simulink model "RBCM_Model"  (R2024b)
settings: Solver=FixedStepAuto  StartTime=0.0  StopTime=10.0  RelTol=1e-3
PreLoadFcn:
  | % NXP_MBDT_S32K3 callback: DO NOT REMOVE
  | mbd_s32k3.common.nxp.model_callbacks.preLoadFcn();
PostLoadFcn:
  | % NXP_MBDT_S32K3 callback: DO NOT REMOVE
  | mbd_s32k3.common.nxp.model_callbacks.postLoadFcn();
InitFcn:
  | % NXP_MBDT_S32K3 callback: DO NOT REMOVE
  | mbd_s32k3.common.nxp.model_callbacks.initFcn();
undefined symbols (not defined in the file or in its folder): AccuFanPwr_hHsd3ch2, BspdPwr_lHsd1ch2, BuzzerPwr_lHsd3ch3, DevicePwr_12v_lHsd1ch1, DevicePwr_hHsd1ch2, DrsPwr_8v_lHsd3ch1, hHsd_Diagnose_AdcBuffer, ILPwr_hHsd1ch1, lHsd_Diagnose_AdcBuffer, LoggerPwr_lHsd1ch3, PumpFan1_hHsd4ch1, PumpFan2_hHsd4ch2, PumpPwr_hHsd3ch1, RGBLED0state, TaillightPwr_lHsd3ch4, TempSensorPwr_lHsd1ch4
libraries: mbd_s32k3_io_library x127, simulink x48, canmsglib x8, mbd_s32k3_communication_library x7, mbd_s32k3_isr_library x6, mbd_s32k3_cdd_library x3, mbd_s32k3_utility_library x1
(part 9 of 10)

== system RBCM_Model/HSD诊断分析子系统/旧模型/HSDh片选执行单元3 ==
  y : Inport
  Data Type Conversion4 : DataTypeConversion  OutDataTypeStr=boolean  SaturateOnIntegerOverflow=off  RndMeth=Floor
  Dio : mbd_s32k3_io_library/Dio  api_func=Dio_WriteChannel  channel=RGBLED0_BLUE  channel_group=No channel groups configured  port=PTB_H  gpioSim=on  text=<binary blob, 15399 chars, not shown>
      settings: SourceProductName=IO Blocks
  wires:
  Data Type Conversion4/1 -> Dio/1
  y/1 -> Data Type Conversion4/1

== system RBCM_Model/HSD诊断分析子系统/旧模型/HSDh片选执行单元4 ==
  y : Inport
  Data Type Conversion4 : DataTypeConversion  OutDataTypeStr=boolean  SaturateOnIntegerOverflow=off  RndMeth=Floor
  Dio : mbd_s32k3_io_library/Dio  api_func=Dio_WriteChannel  channel=RGBLED0_BLUE  channel_group=No channel groups configured  port=PTB_H  gpioSim=on  text=<binary blob, 15399 chars, not shown>
      settings: SourceProductName=IO Blocks
  wires:
  y/1 -> Data Type Conversion4/1
  Data Type Conversion4/1 -> Dio/1

== system RBCM_Model/HSD诊断分析子系统/旧模型/HSDl片选执行单元2 ==
  y : Inport
  Bitwise AND2 : simulink/Logic and Bit Operations/Bitwise Operator  logicop=AND  UseBitMask=on  BitMask=bin2dec('00000001')  BitMaskRealWorld=Stored Integer
      settings: LibrarySourceBlock=|
      | simulink/Quick Insert/Logic and Bit
      | Operations/Bitwise AND
  Bitwise AND3 : simulink/Logic and Bit Operations/Bitwise Operator  logicop=AND  UseBitMask=on  BitMask=bin2dec('00000010')  BitMaskRealWorld=Stored Integer
      settings: LibrarySourceBlock=|
      | simulink/Quick Insert/Logic and Bit
      | Operations/Bitwise AND
  Data Type Conversion : DataTypeConversion  OutDataTypeStr=boolean  SaturateOnIntegerOverflow=off  RndMeth=Floor
  Data Type Conversion1 : DataTypeConversion  OutDataTypeStr=boolean  SaturateOnIntegerOverflow=off  RndMeth=Floor
  Dio : mbd_s32k3_io_library/Dio  api_func=Dio_WriteChannel  channel=RGBLED0_BLUE  channel_group=No channel groups configured  port=PTB_H  gpioSim=on  text=<binary blob, 15399 chars, not shown>
      settings: SourceProductName=IO Blocks
  Dio1 : mbd_s32k3_io_library/Dio  api_func=Dio_WriteChannel  channel=RGBLED0_BLUE  channel_group=No channel groups configured  port=PTB_H  gpioSim=on  text=<binary blob, 15399 chars, not shown>
      settings: SourceProductName=IO Blocks
  Shift Arithmetic1 : ArithShift  BitShiftNumber=1  BitShiftDirection=Right
  Shift Arithmetic2 : ArithShift  BitShiftDirection=Right
  wires:
  Data Type Conversion1/1 -> Dio1/1
  Data Type Conversion/1 -> Dio/1
  y/1 -> Bitwise AND3/1, Bitwise AND2/1
  Shift Arithmetic2/1 -> Data Type Conversion/1
  Bitwise AND3/1 -> Shift Arithmetic1/1
  Bitwise AND2/1 -> Shift Arithmetic2/1
  Shift Arithmetic1/1 -> Data Type Conversion1/1

== system RBCM_Model/HSD诊断分析子系统/旧模型/HSDl片选执行单元3 ==
  y : Inport
  Bitwise AND2 : simulink/Logic and Bit Operations/Bitwise Operator  logicop=AND  UseBitMask=on  BitMask=bin2dec('00000001')  BitMaskRealWorld=Stored Integer
      settings: LibrarySourceBlock=|
      | simulink/Quick Insert/Logic and Bit
      | Operations/Bitwise AND
  Bitwise AND3 : simulink/Logic and Bit Operations/Bitwise Operator  logicop=AND  UseBitMask=on  BitMask=bin2dec('00000010')  BitMaskRealWorld=Stored Integer
      settings: LibrarySourceBlock=|
      | simulink/Quick Insert/Logic and Bit
      | Operations/Bitwise AND
  Data Type Conversion : DataTypeConversion  OutDataTypeStr=boolean  SaturateOnIntegerOverflow=off  RndMeth=Floor
  Data Type Conversion1 : DataTypeConversion  OutDataTypeStr=boolean  SaturateOnIntegerOverflow=off  RndMeth=Floor
  Dio : mbd_s32k3_io_library/Dio  api_func=Dio_WriteChannel  channel=RGBLED0_BLUE  channel_group=No channel groups configured  port=PTB_H  gpioSim=on  text=<binary blob, 15399 chars, not shown>
      settings: SourceProductName=IO Blocks
  Dio1 : mbd_s32k3_io_library/Dio  api_func=Dio_WriteChannel  channel=RGBLED0_BLUE  channel_group=No channel groups configured  port=PTB_H  gpioSim=on  text=<binary blob, 15399 chars, not shown>
      settings: SourceProductName=IO Blocks
  Shift Arithmetic1 : ArithShift  BitShiftNumber=1  BitShiftDirection=Right
  Shift Arithmetic2 : ArithShift  BitShiftDirection=Right
  wires:
  Shift Arithmetic1/1 -> Data Type Conversion1/1
  Bitwise AND2/1 -> Shift Arithmetic2/1
  Bitwise AND3/1 -> Shift Arithmetic1/1
  Shift Arithmetic2/1 -> Data Type Conversion/1
  y/1 -> Bitwise AND2/1, Bitwise AND3/1
  Data Type Conversion/1 -> Dio/1
  Data Type Conversion1/1 -> Dio1/1

== system RBCM_Model/HSD诊断分析子系统/旧模型/HSDl片选执行单元4 ==
  y : Inport
  Bitwise AND2 : simulink/Logic and Bit Operations/Bitwise Operator  logicop=AND  UseBitMask=on  BitMask=bin2dec('00000001')  BitMaskRealWorld=Stored Integer
      settings: LibrarySourceBlock=|
      | simulink/Quick Insert/Logic and Bit
      | Operations/Bitwise AND
  Bitwise AND3 : simulink/Logic and Bit Operations/Bitwise Operator  logicop=AND  UseBitMask=on  BitMask=bin2dec('00000010')  BitMaskRealWorld=Stored Integer
      settings: LibrarySourceBlock=|
      | simulink/Quick Insert/Logic and Bit
      | Operations/Bitwise AND
  Data Type Conversion : DataTypeConversion  OutDataTypeStr=boolean  SaturateOnIntegerOverflow=off  RndMeth=Floor
  Data Type Conversion1 : DataTypeConversion  OutDataTypeStr=boolean  SaturateOnIntegerOverflow=off  RndMeth=Floor
  Dio : mbd_s32k3_io_library/Dio  api_func=Dio_WriteChannel  channel=RGBLED0_BLUE  channel_group=No channel groups configured  port=PTB_H  gpioSim=on  text=<binary blob, 15399 chars, not shown>
      settings: SourceProductName=IO Blocks
  Dio1 : mbd_s32k3_io_library/Dio  api_func=Dio_WriteChannel  channel=RGBLED0_BLUE  channel_group=No channel groups configured  port=PTB_H  gpioSim=on  text=<binary blob, 15399 chars, not shown>
      settings: SourceProductName=IO Blocks
  Shift Arithmetic1 : ArithShift  BitShiftNumber=1  BitShiftDirection=Right
  Shift Arithmetic2 : ArithShift  BitShiftDirection=Right
  wires:
  Data Type Conversion1/1 -> Dio1/1
  Data Type Conversion/1 -> Dio/1
  y/1 -> Bitwise AND3/1, Bitwise AND2/1
  Shift Arithmetic2/1 -> Data Type Conversion/1
  Bitwise AND3/1 -> Shift Arithmetic1/1
  Bitwise AND2/1 -> Shift Arithmetic2/1
  Shift Arithmetic1/1 -> Data Type Conversion1/1

== system RBCM_Model/HSD诊断分析子系统/旧模型/HSDl片选执行单元5 ==
  y : Inport
  Bitwise AND2 : simulink/Logic and Bit Operations/Bitwise Operator  logicop=AND  UseBitMask=on  BitMask=bin2dec('00000001')  BitMaskRealWorld=Stored Integer
      settings: LibrarySourceBlock=|
      | simulink/Quick Insert/Logic and Bit
      | Operations/Bitwise AND
  Bitwise AND3 : simulink/Logic and Bit Operations/Bitwise Operator  logicop=AND  UseBitMask=on  BitMask=bin2dec('00000010')  BitMaskRealWorld=Stored Integer
      settings: LibrarySourceBlock=|
      | simulink/Quick Insert/Logic and Bit
      | Operations/Bitwise AND
  Data Type Conversion : DataTypeConversion  OutDataTypeStr=boolean  SaturateOnIntegerOverflow=off  RndMeth=Floor
  Data Type Conversion1 : DataTypeConversion  OutDataTypeStr=boolean  SaturateOnIntegerOverflow=off  RndMeth=Floor
  Dio : mbd_s32k3_io_library/Dio  api_func=Dio_WriteChannel  channel=RGBLED0_BLUE  channel_group=No channel groups configured  port=PTB_H  gpioSim=on  text=<binary blob, 15399 chars, not shown>
      settings: SourceProductName=IO Blocks
  Dio1 : mbd_s32k3_io_library/Dio  api_func=Dio_WriteChannel  channel=RGBLED0_BLUE  channel_group=No channel groups configured  port=PTB_H  gpioSim=on  text=<binary blob, 15399 chars, not shown>
      settings: SourceProductName=IO Blocks
  Shift Arithmetic1 : ArithShift  BitShiftNumber=1  BitShiftDirection=Right
  Shift Arithmetic2 : ArithShift  BitShiftDirection=Right
  wires:
  Shift Arithmetic1/1 -> Data Type Conversion1/1
  Bitwise AND2/1 -> Shift Arithmetic2/1
  Bitwise AND3/1 -> Shift Arithmetic1/1
  Shift Arithmetic2/1 -> Data Type Conversion/1
  y/1 -> Bitwise AND2/1, Bitwise AND3/1
  Data Type Conversion/1 -> Dio/1
  Data Type Conversion1/1 -> Dio1/1

== system RBCM_Model/HSD诊断分析子系统/旧模型/Subsystem1 ==
  u1 : Inport
  Constant : Constant  Value=0xff  OutDataTypeStr=uint8
  Constant2 : Constant  Value=0  OutDataTypeStr=uint8
  Constant3 : Constant  OutDataTypeStr=uint8
  Constant4 : Constant  Value=2  OutDataTypeStr=uint8
  Gain : Gain  Gain=100
  Multiport Switch : MultiPortSwitch  DataPortOrder=Specify indices  DataPortIndices={0,5,290}  DataPortForDefault=Additional data port  DiagnosticForDefault=Warning  SaturateOnIntegerOverflow=off  InputSameDT=off
  u : Outport
  wires:
  Constant4/1 -> Multiport Switch/4
  Constant3/1 -> Multiport Switch/3
  Constant2/1 -> Multiport Switch/2
  Constant/1 -> Multiport Switch/5
  Multiport Switch/1 -> u/1
  Gain/1 -> Multiport Switch/1
  u1/1 -> Gain/1

== system RBCM_Model/HSD驱动子系统/Subsystem1/HSDh输出控制单元1 ==
  In1 : Inport
  In2 : Inport  Port=2
  Dio : mbd_s32k3_io_library/Dio  api_func=Dio_WriteChannel  channel=RGBLED0_BLUE  channel_group=No channel groups configured  port=PTB_H  gpioSim=on  text=<binary blob, 15399 chars, not shown>
      settings: SourceProductName=IO Blocks
  Dio1 : mbd_s32k3_io_library/Dio  api_func=Dio_WriteChannel  channel=RGBLED0_BLUE  channel_group=No channel groups configured  port=PTB_H  gpioSim=on  text=<binary blob, 15399 chars, not shown>
      settings: SourceProductName=IO Blocks
  wires:
  In2/1 -> Dio1/1
  In1/1 -> Dio/1

== system RBCM_Model/HSD驱动子系统/Subsystem1/HSDh输出控制单元2 ==
  note: PUMP_PWM_CTRL
  In1 : Inport  OutDataTypeStr=uint8
  In2 : Inport  Port=2  OutDataTypeStr=uint8
  Dio : mbd_s32k3_io_library/Dio  api_func=Dio_WriteChannel  channel=RGBLED0_BLUE  channel_group=No channel groups configured  port=PTB_H  gpioSim=on  text=<binary blob, 15399 chars, not shown>
      settings: SourceProductName=IO Blocks
  Dio1 : mbd_s32k3_io_library/Dio  api_func=Dio_WriteChannel  channel=RGBLED0_BLUE  channel_group=No channel groups configured  port=PTB_H  gpioSim=on  text=<binary blob, 15399 chars, not shown>
      settings: SourceProductName=IO Blocks
  wires:
  In2/1 -> Dio1/1
  In1/1 -> Dio/1

== system RBCM_Model/HSD驱动子系统/Subsystem1/HSDh输出控制单元3 ==
  note: FAN1_PWM_CTRL
  In1 : Inport
  In2 : Inport  Port=2
  Dio : mbd_s32k3_io_library/Dio  api_func=Dio_WriteChannel  channel=RGBLED0_BLUE  channel_group=No channel groups configured  port=PTB_H  gpioSim=on  text=<binary blob, 15399 chars, not shown>
      settings: SourceProductName=IO Blocks
  Dio1 : mbd_s32k3_io_library/Dio  api_func=Dio_WriteChannel  channel=RGBLED0_BLUE  channel_group=No channel groups configured  port=PTB_H  gpioSim=on  text=<binary blob, 15399 chars, not shown>
      settings: SourceProductName=IO Blocks
  wires:
  In2/1 -> Dio1/1
  In1/1 -> Dio/1

== system RBCM_Model/HSD驱动子系统/Subsystem1/HSDh输出控制单元4 ==
  note: FAN1_PWM_CTRL
  In1 : Inport
  In2 : Inport  Port=2
  Dio : mbd_s32k3_io_library/Dio  api_func=Dio_WriteChannel  channel=RGBLED0_BLUE  channel_group=No channel groups configured  port=PTB_H  gpioSim=on  text=<binary blob, 15399 chars, not shown>
      settings: SourceProductName=IO Blocks
  Dio1 : mbd_s32k3_io_library/Dio  api_func=Dio_WriteChannel  channel=RGBLED0_BLUE  channel_group=No channel groups configured  port=PTB_H  gpioSim=on  text=<binary blob, 15399 chars, not shown>
      settings: SourceProductName=IO Blocks
  wires:
  In2/1 -> Dio1/1
  In1/1 -> Dio/1

== system RBCM_Model/HSD驱动子系统/Subsystem1/HSDh输出控制单元5 ==
  In1 : Inport
  In2 : Inport  Port=2
  Dio : mbd_s32k3_io_library/Dio  api_func=Dio_WriteChannel  channel=RGBLED0_BLUE  channel_group=No channel groups configured  port=PTB_H  gpioSim=on  text=<binary blob, 15399 chars, not shown>
      settings: SourceProductName=IO Blocks
  Dio1 : mbd_s32k3_io_library/Dio  api_func=Dio_WriteChannel  channel=RGBLED0_BLUE  channel_group=No channel groups configured  port=PTB_H  gpioSim=on  text=<binary blob, 15399 chars, not shown>
      settings: SourceProductName=IO Blocks
  wires:
  In2/1 -> Dio1/1
  In1/1 -> Dio/1

== system RBCM_Model/HSD驱动子系统/Subsystem1/HSDl输出控制单元1 ==
  In1 : Inport
  In2 : Inport  Port=2
  In3 : Inport  Port=3
  In6 : Inport  Port=4
  Dio{,1..3} (4 alike) : mbd_s32k3_io_library/Dio  api_func=Dio_WriteChannel  channel=RGBLED0_BLUE  channel_group=No channel groups configured  port=PTB_H  gpioSim=on  text=<binary blob, 15399 chars, not shown>
      settings: SourceProductName=IO Blocks
  wires:
  In6/1 -> Dio3/1
  In2/1 -> Dio1/1
  In3/1 -> Dio2/1
  In1/1 -> Dio/1

== system RBCM_Model/HSD驱动子系统/Subsystem1/HSDl输出控制单元2 ==
  In1 : Inport
  In2 : Inport  Port=2
  In3 : Inport  Port=3
  In6 : Inport  Port=4
  Dio{,1,3..4} (4 alike) : mbd_s32k3_io_library/Dio  api_func=Dio_WriteChannel  channel=RGBLED0_BLUE  channel_group=No channel groups configured  port=PTB_H  gpioSim=on  text=<binary blob, 15399 chars, not shown>
      settings: SourceProductName=IO Blocks
  wires:
  In1/1 -> Dio/1
  In3/1 -> Dio4/1
  In2/1 -> Dio1/1
  In6/1 -> Dio3/1

== system RBCM_Model/HSD驱动子系统/Subsystem1/HSDl输出控制单元3 ==
  In1 : Inport
  In2 : Inport  Port=2
  In3 : Inport  Port=3
  In6 : Inport  Port=4
  Dio{,1..3} (4 alike) : mbd_s32k3_io_library/Dio  api_func=Dio_WriteChannel  channel=RGBLED0_BLUE  channel_group=No channel groups configured  port=PTB_H  gpioSim=on  text=<binary blob, 15399 chars, not shown>
      settings: SourceProductName=IO Blocks
  wires:
  In6/1 -> Dio3/1
  In2/1 -> Dio1/1
  In3/1 -> Dio2/1
  In1/1 -> Dio/1

== system RBCM_Model/HSD驱动子系统/Subsystem1/HSDl输出控制单元4 ==
  In1 : Inport
  In2 : Inport  Port=2
  In3 : Inport  Port=3
  In6 : Inport  Port=4
  Dio{,1..3} (4 alike) : mbd_s32k3_io_library/Dio  api_func=Dio_WriteChannel  channel=RGBLED0_BLUE  channel_group=No channel groups configured  port=PTB_H  gpioSim=on  text=<binary blob, 15399 chars, not shown>
      settings: SourceProductName=IO Blocks
  wires:
  In1/1 -> Dio/1
  In3/1 -> Dio2/1
  In2/1 -> Dio1/1
  In6/1 -> Dio3/1

== system RBCM_Model/HSD驱动子系统/Subsystem1/HSDl输出控制单元5 ==
  In1 : Inport
  In2 : Inport  Port=2
  In3 : Inport  Port=3
  In6 : Inport  Port=4
  Dio{,1..3} (4 alike) : mbd_s32k3_io_library/Dio  api_func=Dio_WriteChannel  channel=RGBLED0_BLUE  channel_group=No channel groups configured  port=PTB_H  gpioSim=on  text=<binary blob, 15399 chars, not shown>
      settings: SourceProductName=IO Blocks
  wires:
  In6/1 -> Dio3/1
  In2/1 -> Dio1/1
  In3/1 -> Dio2/1
  In1/1 -> Dio/1

== system RBCM_Model/指令报文解码器/Subsystem3/旧模型（放弃） ==
  In1 : Inport  OutDataTypeStr=Bus: Bus_CAN_RX_MESSAG
  CAN Unpack : canmsglib/CAN Unpack  CANdbFile=E:\WUTE\整车CAN通信\E10_240721.dbc  MsgList=(none)  MsgName=PDB_Ctrl  MsgIDType=Extended (29-bit identifier)  MsgIdentifier=514  MsgLength=8  SignalInfo={'PDB_Ctrl_Beep','4','2','LE','unsigned','Standard','0','1','0','0','2';'PDB_Ctrl_DRS','6','2','LE','unsigned','Standard','0','1','0','0','2';'PDB_Ctrl_FAN1','8','8','LE','unsigned','Standard','0','1','0','0','100';'PDB_Ctrl_FAN2','16','8','LE','unsigned','Standard','0','1','0','0','100';'PDB_Ctrl_FAN3','24','8','LE','unsigned','Standard','0','1','0','0','100';'PDB_Ctrl_Pump','2','2','LE','unsigned','Standard','0','1','0','0','2';'PDB_Ctrl_Taillight','0','2','LE','unsigned','Standard','0','1','0','0','2'}  IDPort=off  TimestampPort=off  ErrorPort=off  RemotePort=off  LengthPort=off  StatusPort=off  ApplyMinMax=off
      settings: LibrarySourceBlock=canlib/CAN Unpack  DataFormat=CANdb specified signals
  Chart : Stateflow chart  TreatAsAtomicUnit=on
      settings: PortSchema="{\"entries\":[{\"content\":{\"sides\":[{\"content\":{\"connectorIds\":[\"In1\"]},\"type\":\"ConnectorPlacement.EquallySpacedRectSide\",\"uuid\":\"713ee0ef-c88d-4089-94b4-d4a9f4a2144a\"},{\"content\":{\"connectorIds\":[\"Out2\",\"Out1\"],\"side\":\"RIGHT\"},\"type\":\"ConnectorPlacement.EquallySpacedRectSide\",\"uuid\":\"cedd9109-f959-4345-9ad3-6ca912cd3359\"},{\"content\":{\"side\":\"TOP\"},\"type\":\"ConnectorPlacement.EquallySpacedRectSide\",\"uuid\":\"04e52fa6-1097-4de3-ac45-a6121735278e\"}]},\"type\":\"ConnectorPlacement.EquallySpacedConnector\",\"uuid\":\"ec52044a-9871-4362-8569-ad6e413863bf\"}],\"packageUris\":[\"http://schema.mathworks.com/mf0/Connector/R2020b\"],\"version\":\"1.0\"}"
  Chart1 : Stateflow chart  TreatAsAtomicUnit=on
      settings: PortSchema="{\"entries\":[{\"content\":{\"sides\":[{\"content\":{\"connectorIds\":[\"In1\"]},\"type\":\"ConnectorPlacement.EquallySpacedRectSide\",\"uuid\":\"c3226009-32ac-4581-bd68-d7c78832d05e\"},{\"content\":{\"connectorIds\":[\"Out2\",\"Out1\"],\"side\":\"RIGHT\"},\"type\":\"ConnectorPlacement.EquallySpacedRectSide\",\"uuid\":\"03d88721-aae7-4fe5-8210-7960f8bdfb32\"},{\"content\":{\"side\":\"TOP\"},\"type\":\"ConnectorPlacement.EquallySpacedRectSide\",\"uuid\":\"05beb852-235e-44ab-a3e6-2e32c0da6cde\"}]},\"type\":\"ConnectorPlacement.EquallySpacedConnector\",\"uuid\":\"82dc9e5b-39e8-487e-b276-ca7d7f456cfb\"}],\"packageUris\":[\"http://schema.mathworks.com/mf0/Connector/R2020b\"],\"version\":\"1.0\"}"
  Chart2 : Stateflow chart  TreatAsAtomicUnit=on
      settings: PortSchema="{\"entries\":[{\"content\":{\"sides\":[{\"content\":{\"connectorIds\":[\"In1\"]},\"type\":\"ConnectorPlacement.EquallySpacedRectSide\",\"uuid\":\"713ee0ef-c88d-4089-94b4-d4a9f4a2144a\"},{\"content\":{\"connectorIds\":[\"Out2\",\"Out1\"],\"side\":\"RIGHT\"},\"type\":\"ConnectorPlacement.EquallySpacedRectSide\",\"uuid\":\"cedd9109-f959-4345-9ad3-6ca912cd3359\"},{\"content\":{\"side\":\"TOP\"},\"type\":\"ConnectorPlacement.EquallySpacedRectSide\",\"uuid\":\"04e52fa6-1097-4de3-ac45-a6121735278e\"}]},\"type\":\"ConnectorPlacement.EquallySpacedConnector\",\"uuid\":\"ec52044a-9871-4362-8569-ad6e413863bf\"}],\"packageUris\":[\"http://schema.mathworks.com/mf0/Connector/R2020b\"],\"version\":\"1.0\"}"
  Data Store Write2 : DataStoreWrite  DataStoreName=fan1_pwm_command  IndexOptions=Index vector (dialog)  Indices=1  OutputSizes=1
  Data Store Write4 : DataStoreWrite  DataStoreName=fan2_pwm_command  IndexOptions=Index vector (dialog)  Indices=1  OutputSizes=1
  Data Store Write5 : DataStoreWrite  DataStoreName=fan3_pwm_command  IndexOptions=Index vector (dialog)  Indices=1  OutputSizes=1
  Data Store Write6 : DataStoreWrite  DataStoreName=taillight_pwm_command  IndexOptions=Index vector (dialog)  Indices=1  OutputSizes=1
  Subsystem : Subsystem
  Subsystem1 : Subsystem
  Subsystem2 : Subsystem
  Out1 : Outport
  Out2 : Outport  Port=2
  Out3 : Outport  Port=3
  wires:
  Subsystem2/1(Out1) -> Out3/1
  Subsystem1/1(Out1) -> Out2/1
  Chart2/1(output) -> Subsystem2/1(output)
  Chart1/2(trigger()) -> Subsystem1/Trigger
  Chart1/1(output) -> Subsystem1/1(output)
  CAN Unpack/4 -> Data Store Write4/1
  CAN Unpack/6 -> Chart2/1(input)
  In1/1 -> CAN Unpack/1
  CAN Unpack/2 -> Chart1/1(input)
  CAN Unpack/7 -> Data Store Write6/1
  Subsystem/1(Out1) -> Out1/1
  Chart/1(output) -> Subsystem/1(In1)
  Chart/2(trigger()) -> Subsystem/Trigger
  CAN Unpack/5 -> Data Store Write5/1
  Chart2/2(trigger()) -> Subsystem2/Trigger
  CAN Unpack/3 -> Data Store Write2/1
  CAN Unpack/1 -> Chart/1(input)

== system RBCM_Model/指令报文解码器/Subsystem3/旧模型（放弃）/Subsystem ==
  In1 : Inport
  function : TriggerPort  TriggerType=function-call  VariantControl=Variant
  Add : Sum
  Constant1 : Constant
  Data Store Read : DataStoreRead  DataStoreName=hsd_en_command  IndexOptions=Index vector (dialog)  Indices=1  OutputSizes=1
  Logical Operator2 : Logic  AllPortsSameDT=off  OutDataTypeStr=boolean
  Logical Operator3 : Logic  Operator=NOT  AllPortsSameDT=off  OutDataTypeStr=boolean
  Shift Arithmetic1 : ArithShift  BitShiftNumber=1  BitShiftDirection=Left
  Shift Arithmetic2 : ArithShift  BitShiftNumber=1  BitShiftDirection=Left
  Out1 : Outport  OutDataTypeStr=uint32
  wires:
  Constant1/1 -> Shift Arithmetic1/1
  Add/1 -> Out1/1
  In1/1 -> Shift Arithmetic2/1
  Shift Arithmetic1/1 -> Logical Operator3/1
  Data Store Read/1 -> Logical Operator2/1
  Shift Arithmetic2/1 -> Add/2
  Logical Operator2/1 -> Add/1
  Logical Operator3/1 -> Logical Operator2/2

== system RBCM_Model/指令报文解码器/Subsystem3/旧模型（放弃）/Subsystem1 ==
  output : Inport
  function : TriggerPort  TriggerType=function-call  VariantControl=Variant
  Add : Sum
  Constant1 : Constant
  Data Store Read : DataStoreRead  DataStoreName=hsd_en_command  IndexOptions=Index vector (dialog)  Indices=1  OutputSizes=1
  Logical Operator2 : Logic  AllPortsSameDT=off  OutDataTypeStr=boolean
  Logical Operator3 : Logic  Operator=NOT  AllPortsSameDT=off  OutDataTypeStr=boolean
  Shift Arithmetic1 : ArithShift  BitShiftNumber=2  BitShiftDirection=Left
  Shift Arithmetic2 : ArithShift  BitShiftNumber=2  BitShiftDirection=Left
  Out1 : Outport  OutDataTypeStr=uint32
  wires:
  Logical Operator3/1 -> Logical Operator2/2
  Logical Operator2/1 -> Add/1
  Shift Arithmetic2/1 -> Add/2
  Data Store Read/1 -> Logical Operator2/1
  Shift Arithmetic1/1 -> Logical Operator3/1
  output/1 -> Shift Arithmetic2/1
  Add/1 -> Out1/1
  Constant1/1 -> Shift Arithmetic1/1

== system RBCM_Model/指令报文解码器/Subsystem3/旧模型（放弃）/Subsystem2 ==
  output : Inport
  function : TriggerPort  TriggerType=function-call  VariantControl=Variant
  Add : Sum
  Constant1 : Constant
  Data Store Read : DataStoreRead  DataStoreName=hsd_en_command  IndexOptions=Index vector (dialog)  Indices=1  OutputSizes=1
  Logical Operator2 : Logic  AllPortsSameDT=off  OutDataTypeStr=boolean
  Logical Operator3 : Logic  Operator=NOT  AllPortsSameDT=off  OutDataTypeStr=boolean
  Shift Arithmetic1 : ArithShift  BitShiftNumber=3  BitShiftDirection=Left
  Shift Arithmetic2 : ArithShift  BitShiftNumber=3  BitShiftDirection=Left
  Out1 : Outport  OutDataTypeStr=uint32
  wires:
  Constant1/1 -> Shift Arithmetic1/1
  Add/1 -> Out1/1
  output/1 -> Shift Arithmetic2/1
  Shift Arithmetic1/1 -> Logical Operator3/1
  Data Store Read/1 -> Logical Operator2/1
  Shift Arithmetic2/1 -> Add/2
  Logical Operator2/1 -> Add/1
  Logical Operator3/1 -> Logical Operator2/2

== matlab function RBCM_Model/Subsystem5/Subsystem/MATLAB Function ==
  data: y output Bus: Bus_Hsd_Drive_Commands
function y = fcn
y.DevicePwr_12v_lHsd1ch1 = 1;
y.BspdPwr_lHsd1ch2 = 1;
y.LoggerPwr_lHsd1ch3 = 1;
y.TempSensorPwr_lHsd1ch4 = 1;

y.DevicePwr_12v_lHsd2ch1 = 1;
y.VcuPwr_lHsd2ch2 = 1;
y.Fireon_Pwr_lHsd2ch3 = 1;
y.DsbdPwr_lHsd2ch4 = 1;

y.DrsPwr_8v_lHsd3ch1 = 1;
y.DevicePwr_lHsd3ch2 = 1;
y.BuzzerPwr_lHsd3ch3 = 1;
y.TaillightPwr_lHsd3ch4 = 1;

y.DevicePwr_5v_lHsd4ch1 = 1;
y.AccuUbr_lHsd4ch2 = 1;
y.AccuPwr_lHsd4ch3 = 1;
y.BduPwr_lHsd4ch4 = 1;

y.DevicePwr_5v_lHsd5ch1 = 1;
y.McuUbr_lHsd5ch2 = 1;
y.EnergeMeterPwr_lHsd5ch3 = 1;
y.TsalrPwr_lHsd5ch4 = 1;


y.ILPwr_hHsd1ch1 = 1;
y.DevicePwr_hHsd1ch2 = 1;

y.VcuUbr_hHsd2ch1 = 1;
y.Device_hHsd2ch2 = 1;

y.PumpPwr_hHsd3ch1 = 1;
y.AccuFanPwr_hHsd3ch2 = 1;

y.PumpFan1_hHsd4ch1 = 1;
y.PumpFan2_hHsd4ch2 = 1;

y.DevicePwr_hHsd5ch1 = 1;
y.DevicePwr_hHsd5ch2 = 1;

y.DevicePwr_hHsd6ch1 = 1;
y.DevicePwr_hHsd6ch2 = 1;

== stateflow chart RBCM_Model/Subsystem7/Chart2 ==
  state A
  state A1
  (default) -> A
  A -> A1
  A1 -> A
  data: A output boolean [0..1]

== matlab function RBCM_Model/HSD诊断分析子系统/触发器1 ==
  data: y output uint8; counter input uint8; u2 input uint8
  events: fcncall output FUNCTION_CALL_EVENT
function y = fcn(counter,u2)

% 函数内部声明 可持续类型变量 output
persistent i
persistent output  
% 首先要判断persistent声明的变量是否是空
if isempty(i)
    i  = 0;
end
if isempty(output)
    output  = 0;
end

% 自递增
i=i+1;
output=output+1;

%分频计数值溢出
if i>=counter
    %输出值溢出
    if output>=u2
        output=0;
    end

    %输出值
    y = uint8(output);

    %生成触发，触发ADC采集
    fcncall;

    i=0;
else
    y=uint8(output);    %不生成触发
end

end

== matlab function RBCM_Model/HSD诊断分析子系统/触发器11 ==
  data: y output uint8; counter input uint8; u2 input uint8
  events: fcncall output FUNCTION_CALL_EVENT
function y = fcn(counter,u2)

% 函数内部声明 可持续类型变量 output
persistent i
persistent output  
% 首先要判断persistent声明的变量是否是空
if isempty(i)
    i  = 0;
end
if isempty(output)
    output  = 0;
end

% 自递增
i=i+1;
output=output+1;

%分频计数值溢出
if i>=counter
    %输出值溢出
    if output>=u2
        output=0;
    end

    %输出值
    y = uint8(output);

    %生成触发，触发ADC采集
    fcncall;

    i=0;
else
    y=uint8(output);    %不生成触发
end

end

== matlab function RBCM_Model/HSD诊断分析子系统/数据转存单元11 ==
  data: index input uint8; u input uint16; y1 output uint16; y2 output uint16
function [y1, y2] = fcn2(index, u)

% 函数内部声明 可持续类型变量
persistent Y1 Y2
% 首先要判断persistent声明的变量是否是空
if isempty(Y1)
    Y1=uint16(0);
    Y2=uint16(0);
end

if index==0
    y1=u;
    y2=Y2;
elseif index==1
    y1=Y1;
    y2=u;
else
    y1=Y1;
    y2=Y2;
end

Y1=y1;
Y2=y2;

end

== matlab function RBCM_Model/HSD诊断分析子系统/旧模型/数据转存单元2 ==
  data: index input uint8; u input uint8; y1 output uint8; y2 output uint8; y3 output uint8; y4 output uint8
function [y1, y2, y3, y4] = fcn2(index, u)

% 函数内部声明 可持续类型变量
persistent Y1 Y2 Y3 Y4
% 首先要判断persistent声明的变量是否是空
if isempty(Y1)
    Y1=uint8(0);
    Y2=uint8(0);
    Y3=uint8(0);
    Y4=uint8(0);
end

if index==0
    y1=u;
    y2=Y2;
    y3=Y3;
    y4=Y4;
elseif index==1
    y1=Y1;
    y2=u;
    y3=Y3;
    y4=Y4;
elseif index==2
    y1=Y1;
    y2=Y2;
    y3=u;
    y4=Y4;
elseif index==3
    y1=Y1;
    y2=Y2;
    y3=Y3;
    y4=u;
else
    y1=Y1;
    y2=Y2;
    y3=Y3;
    y4=Y4;
end

Y1=y1;
Y2=y2;
Y3=y3;
Y4=y4;

end

== matlab function RBCM_Model/HSD诊断分析子系统/旧模型/触发器2 ==
  data: y output uint8; counter input uint8; u2 input uint8
  events: fcncall output FUNCTION_CALL_EVENT
function y = fcn(counter,u2)

% 函数内部声明 可持续类型变量 output
persistent i
persistent output  
% 首先要判断persistent声明的变量是否是空
if isempty(i)
    i  = 0;
end
if isempty(output)
    output  = 0;
end

% 自递增
i=i+1;
output=output+1;

%分频计数值溢出
if i>=counter
    %输出值溢出
    if output>=u2
        output=0;
    end

    %输出值
    y = uint8(output);

    %生成触发，触发ADC采集
    fcncall;

    i=0;
else
    y=uint8(output);    %不生成触发
end

end

== matlab function RBCM_Model/HSD诊断分析子系统/旧模型/数据转存单元3 ==
  data: index input uint8; u input uint8; y1 output uint8; y2 output uint8; y3 output uint8; y4 output uint8
function [y1, y2, y3, y4] = fcn2(index, u)

% 函数内部声明 可持续类型变量
persistent Y1 Y2 Y3 Y4
% 首先要判断persistent声明的变量是否是空
if isempty(Y1)
    Y1=uint8(0);
    Y2=uint8(0);
    Y3=uint8(0);
    Y4=uint8(0);
end

if index==0
    y1=u;
    y2=Y2;
    y3=Y3;
    y4=Y4;
elseif index==1
    y1=Y1;
    y2=u;
    y3=Y3;
    y4=Y4;
elseif index==2
    y1=Y1;
    y2=Y2;
    y3=u;
    y4=Y4;
elseif index==3
    y1=Y1;
    y2=Y2;
    y3=Y3;
    y4=u;
else
    y1=Y1;
    y2=Y2;
    y3=Y3;
    y4=Y4;
end

Y1=y1;
Y2=y2;
Y3=y3;
Y4=y4;

end

== matlab function RBCM_Model/HSD诊断分析子系统/旧模型/触发器3 ==
  data: y output uint8; counter input uint8; u2 input uint8
  events: fcncall output FUNCTION_CALL_EVENT
function y = fcn(counter,u2)

% 函数内部声明 可持续类型变量 output
persistent i
persistent output  
% 首先要判断persistent声明的变量是否是空
if isempty(i)
    i  = 0;
end
if isempty(output)
    output  = 0;
end

% 自递增
i=i+1;
output=output+1;

%分频计数值溢出
if i>=counter
    %输出值溢出
    if output>=u2
        output=0;
    end

    %输出值
    y = uint8(output);

    %生成触发，触发ADC采集
    fcncall;

    i=0;
else
    y=uint8(output);    %不生成触发
end

end

== matlab function RBCM_Model/HSD诊断分析子系统/旧模型/数据转存单元4 ==
  data: index input uint8; u input uint8; y1 output uint8; y2 output uint8; y3 output uint8; y4 output uint8
function [y1, y2, y3, y4] = fcn2(index, u)

% 函数内部声明 可持续类型变量
persistent Y1 Y2 Y3 Y4
% 首先要判断persistent声明的变量是否是空
if isempty(Y1)
    Y1=uint8(0);
    Y2=uint8(0);
    Y3=uint8(0);
    Y4=uint8(0);
end

if index==0
    y1=u;
    y2=Y2;
    y3=Y3;
    y4=Y4;
elseif index==1
    y1=Y1;
    y2=u;
    y3=Y3;
    y4=Y4;
elseif index==2
    y1=Y1;
    y2=Y2;
    y3=u;
    y4=Y4;
elseif index==3
    y1=Y1;
    y2=Y2;
    y3=Y3;
    y4=u;
else
    y1=Y1;
    y2=Y2;
    y3=Y3;
    y4=Y4;
end

Y1=y1;
Y2=y2;
Y3=y3;
Y4=y4;

end

== matlab function RBCM_Model/HSD诊断分析子系统/旧模型/触发器4 ==
  data: y output uint8; counter input uint8; u2 input uint8
  events: fcncall output FUNCTION_CALL_EVENT
function y = fcn(counter,u2)

% 函数内部声明 可持续类型变量 output
persistent i
persistent output  
% 首先要判断persistent声明的变量是否是空
if isempty(i)
    i  = 0;
end
if isempty(output)
    output  = 0;
end

% 自递增
i=i+1;
output=output+1;

%分频计数值溢出
if i>=counter
    %输出值溢出
    if output>=u2
        output=0;
    end

    %输出值
    y = uint8(output);

    %生成触发，触发ADC采集
    fcncall;

    i=0;
else
    y=uint8(output);    %不生成触发
end

end

== matlab function RBCM_Model/HSD诊断分析子系统/旧模型/数据转存单元5 ==
  data: index input uint8; u input uint8; y1 output uint8; y2 output uint8; y3 output uint8; y4 output uint8
function [y1, y2, y3, y4] = fcn2(index, u)

% 函数内部声明 可持续类型变量
persistent Y1 Y2 Y3 Y4
% 首先要判断persistent声明的变量是否是空
if isempty(Y1)
    Y1=uint8(0);
    Y2=uint8(0);
    Y3=uint8(0);
    Y4=uint8(0);
end

if index==0
    y1=u;
    y2=Y2;
    y3=Y3;
    y4=Y4;
elseif index==1
    y1=Y1;
    y2=u;
    y3=Y3;
    y4=Y4;
elseif index==2
    y1=Y1;
    y2=Y2;
    y3=u;
    y4=Y4;
elseif index==3
    y1=Y1;
    y2=Y2;
    y3=Y3;
    y4=u;
else
    y1=Y1;
    y2=Y2;
    y3=Y3;
    y4=Y4;
end

Y1=y1;
Y2=y2;
Y3=y3;
Y4=y4;

end

== matlab function RBCM_Model/HSD诊断分析子系统/旧模型/触发器5 ==
  data: y output uint8; counter input uint8; u2 input uint8
  events: fcncall output FUNCTION_CALL_EVENT
function y = fcn(counter,u2)

% 函数内部声明 可持续类型变量 output
persistent i
persistent output  
% 首先要判断persistent声明的变量是否是空
if isempty(i)
    i  = 0;
end
if isempty(output)
    output  = 0;
end

% 自递增
i=i+1;
output=output+1;

%分频计数值溢出
if i>=counter
    %输出值溢出
    if output>=u2
        output=0;
    end

    %输出值
    y = uint8(output);

    %生成触发，触发ADC采集
    fcncall;

    i=0;
else
    y=uint8(output);    %不生成触发
end

end

== matlab function RBCM_Model/HSD诊断分析子系统/旧模型/数据转存单元6 ==
  data: index input uint8; u input uint8; y1 output uint8; y2 output uint8
function [y1, y2] = fcn2(index, u)

% 函数内部声明 可持续类型变量
persistent Y1 Y2
% 首先要判断persistent声明的变量是否是空
if isempty(Y1)
    Y1=uint8(0);
    Y2=uint8(0);
end

if index==0
    y1=u;
    y2=Y2;
elseif index==1
    y1=Y1;
    y2=u;
else
    y1=Y1;
    y2=Y2;
end

Y1=y1;
Y2=y2;

end

== matlab function RBCM_Model/HSD诊断分析子系统/旧模型/触发器6 ==
  data: y output uint8; counter input uint8; u2 input uint8
  events: fcncall output FUNCTION_CALL_EVENT
function y = fcn(counter,u2)

% 函数内部声明 可持续类型变量 output
persistent i
persistent output  
% 首先要判断persistent声明的变量是否是空
if isempty(i)
    i  = 0;
end
if isempty(output)
    output  = 0;
end

% 自递增
i=i+1;
output=output+1;

%分频计数值溢出
if i>=counter
    %输出值溢出
    if output>=u2
        output=0;
    end

    %输出值
    y = uint8(output);

    %生成触发，触发ADC采集
    fcncall;

    i=0;
else
    y=uint8(output);    %不生成触发
end

end

== matlab function RBCM_Model/HSD诊断分析子系统/旧模型/数据转存单元7 ==
  data: index input uint8; u input uint8; y1 output uint8; y2 output uint8
function [y1, y2] = fcn2(index, u)

% 函数内部声明 可持续类型变量
persistent Y1 Y2
% 首先要判断persistent声明的变量是否是空
if isempty(Y1)
    Y1=uint8(0);
    Y2=uint8(0);
end

if index==0
    y1=u;
    y2=Y2;
elseif index==1
    y1=Y1;
    y2=u;
else
    y1=Y1;
    y2=Y2;
end

Y1=y1;
Y2=y2;

end

== matlab function RBCM_Model/HSD诊断分析子系统/旧模型/触发器7 ==
  data: y output uint8; counter input uint8; u2 input uint8
  events: fcncall output FUNCTION_CALL_EVENT
function y = fcn(counter,u2)

% 函数内部声明 可持续类型变量 output
persistent i
persistent output  
% 首先要判断persistent声明的变量是否是空
if isempty(i)
    i  = 0;
end
if isempty(output)
    output  = 0;
end

% 自递增
i=i+1;
output=output+1;

%分频计数值溢出
if i>=counter
    %输出值溢出
    if output>=u2
        output=0;
    end

    %输出值
    y = uint8(output);

    %生成触发，触发ADC采集
    fcncall;

    i=0;
else
    y=uint8(output);    %不生成触发
end

end

== matlab function RBCM_Model/HSD诊断分析子系统/旧模型/数据转存单元8 ==
  data: index input uint8; u input uint8; y1 output uint8; y2 output uint8
function [y1, y2] = fcn2(index, u)

% 函数内部声明 可持续类型变量
persistent Y1 Y2
% 首先要判断persistent声明的变量是否是空
if isempty(Y1)
    Y1=uint8(0);
    Y2=uint8(0);
end

if index==0
    y1=u;
    y2=Y2;
elseif index==1
    y1=Y1;
    y2=u;
else
    y1=Y1;
    y2=Y2;
end

Y1=y1;
Y2=y2;

end

== matlab function RBCM_Model/HSD诊断分析子系统/旧模型/触发器8 ==
  data: y output uint8; counter input uint8; u2 input uint8
  events: fcncall output FUNCTION_CALL_EVENT
function y = fcn(counter,u2)

% 函数内部声明 可持续类型变量 output
persistent i
persistent output  
% 首先要判断persistent声明的变量是否是空
if isempty(i)
    i  = 0;
end
if isempty(output)
    output  = 0;
end

% 自递增
i=i+1;
output=output+1;

%分频计数值溢出
if i>=counter
    %输出值溢出
    if output>=u2
        output=0;
    end

    %输出值
    y = uint8(output);

    %生成触发，触发ADC采集
    fcncall;

    i=0;
else
    y=uint8(output);    %不生成触发
end

end

== matlab function RBCM_Model/HSD诊断分析子系统/诊断数据转存单元1 ==
  data: index input uint8; u input uint16; y1 output uint16; y2 output uint16; y3 output uint16; y4 output uint16
function [y1, y2, y3, y4] = fcn2(index, u)

% 函数内部声明 可持续类型变量
persistent Y1 Y2 Y3 Y4
% 首先要判断persistent声明的变量是否是空
if isempty(Y1)
    Y1=uint16(0);
    Y2=uint16(0);
    Y3=uint16(0);
    Y4=uint16(0);
end

if index==0
    y1=u;
    y2=Y2;
    y3=Y3;
    y4=Y4;
elseif index==1
    y1=Y1;
    y2=u;
    y3=Y3;
    y4=Y4;
elseif index==2
    y1=Y1;
    y2=Y2;
    y3=u;
    y4=Y4;
elseif index==3
    y1=Y1;
    y2=Y2;
    y3=Y3;
    y4=u;
else
    y1=Y1;
    y2=Y2;
    y3=Y3;
    y4=Y4;
end

Y1=y1;
Y2=y2;
Y3=y3;
Y4=y4;

end

== matlab function RBCM_Model/HSD诊断分析子系统/旧模型/数据转存单元9 ==
  data: index input uint8; u input uint8; y1 output uint8; y2 output uint8
function [y1, y2] = fcn2(index, u)

% 函数内部声明 可持续类型变量
persistent Y1 Y2
% 首先要判断persistent声明的变量是否是空
if isempty(Y1)
    Y1=uint8(0);
    Y2=uint8(0);
end

if index==0
    y1=u;
    y2=Y2;
elseif index==1
    y1=Y1;
    y2=u;
else
    y1=Y1;
    y2=Y2;
end

Y1=y1;
Y2=y2;

end

== matlab function RBCM_Model/HSD诊断分析子系统/旧模型/触发器9 ==
  data: y output uint8; counter input uint8; u2 input uint8
  events: fcncall output FUNCTION_CALL_EVENT
function y = fcn(counter,u2)

% 函数内部声明 可持续类型变量 output
persistent i
persistent output  
% 首先要判断persistent声明的变量是否是空
if isempty(i)
    i  = 0;
end
if isempty(output)
    output  = 0;
end

% 自递增
i=i+1;
output=output+1;

%分频计数值溢出
if i>=counter
    %输出值溢出
    if output>=u2
        output=0;
    end

    %输出值
    y = uint8(output);

    %生成触发，触发ADC采集
    fcncall;

    i=0;
else
    y=uint8(output);    %不生成触发
end

end

== matlab function RBCM_Model/HSD诊断数据抓取与发送(不启用)/HSD组轮询单元 ==
  data: u input; y output
  events: fcncall output FUNCTION_CALL_EVENT
function y  = fcn(u)

% 函数内部声明 可持续类型变量
persistent group
% 首先要判断persistent声明的变量是否是空
if isempty(group)
    group=0;    %基0始
end

%计数值溢出
if group>=u
    %输出值
    group=0;
end

y = uint8(group);
%生成触发，触发ADC采集
fcncall;

% 自递增
group=group+1;

end

== stateflow chart RBCM_Model/核心状态信息发送/Chart1 ==
  state A
  state A1
  (default) -> A
  A -> A1
  A1 -> A
  data: A output boolean [0..1]

== matlab function RBCM_Model/HSD诊断分析子系统/错误码转存单元10 ==
  data: index input uint8; u input uint8; y1 output uint8; y2 output uint8; y3 output uint8; y4 output uint8
function [y1, y2, y3, y4] = fcn2(index, u)

% 函数内部声明 可持续类型变量
persistent Y1 Y2 Y3 Y4
% 首先要判断persistent声明的变量是否是空
if isempty(Y1)
    Y1=uint8(0);
    Y2=uint8(0);
    Y3=uint8(0);
    Y4=uint8(0);
end

if index==0
    y1=u;
    y2=Y2;
    y3=Y3;
    y4=Y4;
elseif index==1
    y1=Y1;
    y2=u;
    y3=Y3;
    y4=Y4;
elseif index==2
    y1=Y1;
    y2=Y2;
    y3=u;
    y4=Y4;
elseif index==3
    y1=Y1;
    y2=Y2;
    y3=Y3;
    y4=u;
else
    y1=Y1;
    y2=Y2;
    y3=Y3;
    y4=Y4;
end

Y1=y1;
Y2=y2;
Y3=y3;
Y4=y4;

end

== matlab function RBCM_Model/HSD诊断分析子系统/数据转存单元1 ==
  data: index input uint8; u input uint8; y1 output uint8; y2 output uint8
function [y1, y2] = fcn2(index, u)

% 函数内部声明 可持续类型变量
persistent Y1 Y2
% 首先要判断persistent声明的变量是否是空
if isempty(Y1)
    Y1=uint8(0);
    Y2=uint8(0);
end

if index==0
    y1=u;
    y2=Y2;
elseif index==1
    y1=Y1;
    y2=u;
else
    y1=Y1;
    y2=Y2;
end

Y1=y1;
Y2=y2;

end

== stateflow chart RBCM_Model/指令报文解码器/Subsystem3/旧模型（放弃）/Chart ==
  state close
    output=1;
  state open
    output=0;
  (default) -> close
  close -> open : [input==1]{trigger;}
  open -> close : [input==2]{trigger;}
  data: input input uint8; output output uint32
  events: trigger output FUNCTION_CALL_EVENT

== matlab function RBCM_Model/HsdDriveCommand Struct1 ==
  data: HsdDriveCommandsInit output Bus: Bus_Hsd_Drive_Commands
function HsdDriveCommandsInit = fcn

HsdDriveCommandsInit.DevicePwr_12v_lHsd1ch1 = uint8(1);
HsdDriveCommandsInit.BspdPwr_lHsd1ch2 = uint8(1);
HsdDriveCommandsInit.LoggerPwr_lHsd1ch3 = uint8(1);
HsdDriveCommandsInit.TempSensorPwr_lHsd1ch4 = uint8(1);

HsdDriveCommandsInit.DevicePwr_12v_lHsd2ch1 = uint8(1);
HsdDriveCommandsInit.VcuPwr_lHsd2ch2 = uint8(1);
HsdDriveCommandsInit.Fireon_Pwr_lHsd2ch3 = uint8(1);
HsdDriveCommandsInit.DsbdPwr_lHsd2ch4 = uint8(1);

HsdDriveCommandsInit.DrsPwr_8v_lHsd3ch1 = uint8(1);
HsdDriveCommandsInit.DevicePwr_lHsd3ch2 = uint8(1);
HsdDriveCommandsInit.BuzzerPwr_lHsd3ch3 = uint8(1);
HsdDriveCommandsInit.TaillightPwr_lHsd3ch4 = uint8(1);

HsdDriveCommandsInit.DevicePwr_5v_lHsd4ch1 = uint8(1);
HsdDriveCommandsInit.AccuUbr_lHsd4ch2 = uint8(1);
HsdDriveCommandsInit.AccuPwr_lHsd4ch3 = uint8(1);
HsdDriveCommandsInit.BduPwr_lHsd4ch4 = uint8(1);

HsdDriveCommandsInit.DevicePwr_5v_lHsd5ch1 = uint8(1);
HsdDriveCommandsInit.McuUbr_lHsd5ch2 = uint8(1);
HsdDriveCommandsInit.EnergeMeterPwr_lHsd5ch3 = uint8(1);
HsdDriveCommandsInit.TsalrPwr_lHsd5ch4 = uint8(1);


HsdDriveCommandsInit.ILPwr_hHsd1ch1 = uint8(1);
HsdDriveCommandsInit.DevicePwr_hHsd1ch2 = uint8(1);

HsdDriveCommandsInit.VcuUbr_hHsd2ch1 = uint8(1);
HsdDriveCommandsInit.Device_hHsd2ch2 = uint8(1);

HsdDriveCommandsInit.PumpPwr_hHsd3ch1 = uint8(1);
HsdDriveCommandsInit.AccuFanPwr_hHsd3ch2 = uint8(1);

HsdDriveCommandsInit.PumpFan1_hHsd4ch1 = uint8(1);
HsdDriveCommandsInit.PumpFan2_hHsd4ch2 = uint8(1);

HsdDriveCommandsInit.DevicePwr_hHsd5ch1 = uint8(1);
HsdDriveCommandsInit.DevicePwr_hHsd5ch2 = uint8(1);

HsdDriveCommandsInit.DevicePwr_hHsd6ch1 = uint8(1);
HsdDriveCommandsInit.DevicePwr_hHsd6ch2 = uint8(1);

== matlab function RBCM_Model/HSD诊断分析子系统/旧模型/数据转存单元1 ==
  data: index input uint8; u input uint8; y1 output uint8; y2 output uint8
function [y1, y2] = fcn2(index, u)

% 函数内部声明 可持续类型变量
persistent Y1 Y2
% 首先要判断persistent声明的变量是否是空
if isempty(Y1)
    Y1=uint8(0);
    Y2=uint8(0);
end

if index==0
    y1=u;
    y2=Y2;
elseif index==1
    y1=Y1;
    y2=u;
else
    y1=Y1;
    y2=Y2;
end

Y1=y1;
Y2=y2;

end

== matlab function RBCM_Model/HSD诊断分析子系统/旧模型/数据转存单元11 ==
  data: index input uint8; u input uint8; y1 output uint8; y2 output uint8
function [y1, y2] = fcn2(index, u)

% 函数内部声明 可持续类型变量
persistent Y1 Y2
% 首先要判断persistent声明的变量是否是空
if isempty(Y1)
    Y1=uint8(0);
    Y2=uint8(0);
end

if index==0
    y1=u;
    y2=Y2;
elseif index==1
    y1=Y1;
    y2=u;
else
    y1=Y1;
    y2=Y2;
end

Y1=y1;
Y2=y2;

end

== matlab function RBCM_Model/输出3s初始化/MATLAB Function ==
  data: u1 input; y output; u2 input
function y = fcn(u1, u2)

% 函数内部声明 可持续类型变量 output
persistent i
% 首先要判断persistent声明的变量是否是空
if isempty(i)
    i  = 0;
end

if i<3
    y=u1;
    i=i+1;
else
    y=u2;
end

end

== matlab function RBCM_Model/Subsystem2/Add '\r\n'2 ==
  data: u input; y output
function y = fcn(u)

y = [u 10 13];

== matlab function RBCM_Model/Subsystem2/MATLAB Function ==
  data: temp1 input; y output string; temp2 input
function y = fcn(temp1, temp2)

%双引号
dquotes = 34;
%冒号
colon = 58;
%逗号
comma = 44;


s1 = abs('temp1');
s2 = abs('temp2');

%{"key1":100,"key2":20}
%{:123 }:125 ":34 ::58 ,:44
y = [123 34 s1 34 58 temp1 44 34 s1 34 58 temp2 125];

== stateflow chart RBCM_Model/指令报文解码器/Subsystem3/旧模型（放弃）/Chart1 ==
  state close
    output=1;
  state open
    output=0;
  (default) -> close
  close -> open : [input==1]{trigger;}
  open -> close : [input==2]{trigger;}
  data: input input uint8; output output uint32
  events: trigger output FUNCTION_CALL_EVENT

== matlab function RBCM_Model/MATLAB Function ==
  data: DiagnoseValueStruct output Bus: Bus_Hsd_Diagnose_Values
function DiagnoseValueStruct = fcn

DiagnoseValueStruct.DevicePwr_12v_lHsd1ch1 = uint16(0);
DiagnoseValueStruct.BspdPwr_lHsd1ch2 = uint16(0);
DiagnoseValueStruct.LoggerPwr_lHsd1ch3 = uint16(0);
DiagnoseValueStruct.TempSensorPwr_lHsd1ch4 = uint16(0);

DiagnoseValueStruct.DevicePwr_12v_lHsd2ch1 = uint16(0);
DiagnoseValueStruct.VcuPwr_lHsd2ch2 = uint16(0);
DiagnoseValueStruct.Fireon_Pwr_lHsd2ch3 = uint16(0);
DiagnoseValueStruct.DsbdPwr_lHsd2ch4 = uint16(0);

DiagnoseValueStruct.DrsPwr_8v_lHsd3ch1 = uint16(0);
DiagnoseValueStruct.DevicePwr_lHsd3ch2 = uint16(0);
DiagnoseValueStruct.BuzzerPwr_lHsd3ch3 = uint16(0);
DiagnoseValueStruct.TaillightPwr_lHsd3ch4 = uint16(0);

DiagnoseValueStruct.DevicePwr_5v_lHsd4ch1 = uint16(0);
DiagnoseValueStruct.AccuUbr_lHsd4ch2 = uint16(0);
DiagnoseValueStruct.AccuPwr_lHsd4ch3 = uint16(0);
DiagnoseValueStruct.BduPwr_lHsd4ch4 = uint16(0);

DiagnoseValueStruct.DevicePwr_5v_lHsd5ch1 = uint16(0);
DiagnoseValueStruct.McuUbr_lHsd5ch2 = uint16(0);
DiagnoseValueStruct.EnergeMeterPwr_lHsd5ch3 = uint16(0);
DiagnoseValueStruct.TsalrPwr_lHsd5ch4 = uint16(0);


DiagnoseValueStruct.ILPwr_hHsd1ch1 = uint16(0);
DiagnoseValueStruct.DevicePwr_hHsd1ch2 = uint16(0);

DiagnoseValueStruct.VcuUbr_hHsd2ch1 = uint16(0);
DiagnoseValueStruct.Device_hHsd2ch2 = uint16(0);

DiagnoseValueStruct.PumpPwr_hHsd3ch1 = uint16(0);
DiagnoseValueStruct.AccuFanPwr_hHsd3ch2 = uint16(0);

DiagnoseValueStruct.PumpFan1_hHsd4ch1 = uint16(0);
DiagnoseValueStruct.PumpFan2_hHsd4ch2 = uint16(0);

DiagnoseValueStruct.DevicePwr_hHsd5ch1 = uint16(0);
DiagnoseValueStruct.DevicePwr_hHsd5ch2 = uint16(0);

DiagnoseValueStruct.DevicePwr_hHsd6ch1 = uint16(0);
DiagnoseValueStruct.DevicePwr_hHsd6ch2 = uint16(0);

== matlab function RBCM_Model/MATLAB Function1 ==
  data: DiagnoseResultStruct output Bus: Bus_Hsd_Diagnose_Results
function DiagnoseResultStruct = fcn
DiagnoseResultStruct.DevicePwr_12v_lHsd1ch1 = uint8(0);
DiagnoseResultStruct.BspdPwr_lHsd1ch2 = uint8(0);
DiagnoseResultStruct.LoggerPwr_lHsd1ch3 = uint8(0);
DiagnoseResultStruct.TempSensorPwr_lHsd1ch4 = uint8(0);

DiagnoseResultStruct.DevicePwr_12v_lHsd2ch1 = uint8(0);
DiagnoseResultStruct.VcuPwr_lHsd2ch2 = uint8(0);
DiagnoseResultStruct.Fireon_Pwr_lHsd2ch3 = uint8(0);
DiagnoseResultStruct.DsbdPwr_lHsd2ch4 = uint8(0);

DiagnoseResultStruct.DrsPwr_8v_lHsd3ch1 = uint8(0);
DiagnoseResultStruct.DevicePwr_lHsd3ch2 = uint8(0);
DiagnoseResultStruct.BuzzerPwr_lHsd3ch3 = uint8(0);
DiagnoseResultStruct.TaillightPwr_lHsd3ch4 = uint8(0);

DiagnoseResultStruct.DevicePwr_5v_lHsd4ch1 = uint8(0);
DiagnoseResultStruct.AccuUbr_lHsd4ch2 = uint8(0);
DiagnoseResultStruct.AccuPwr_lHsd4ch3 = uint8(0);
DiagnoseResultStruct.BduPwr_lHsd4ch4 = uint8(0);

DiagnoseResultStruct.DevicePwr_5v_lHsd5ch1 = uint8(0);
DiagnoseResultStruct.McuUbr_lHsd5ch2 = uint8(0);
DiagnoseResultStruct.EnergeMeterPwr_lHsd5ch3 = uint8(0);
DiagnoseResultStruct.TsalrPwr_lHsd5ch4 = uint8(0);


DiagnoseResultStruct.ILPwr_hHsd1ch1 = uint8(0);
DiagnoseResultStruct.DevicePwr_hHsd1ch2 = uint8(0);

DiagnoseResultStruct.VcuUbr_hHsd2ch1 = uint8(0);
DiagnoseResultStruct.Device_hHsd2ch2 = uint8(0);

DiagnoseResultStruct.PumpPwr_hHsd3ch1 = uint8(0);
DiagnoseResultStruct.AccuFanPwr_hHsd3ch2 = uint8(0);

DiagnoseResultStruct.PumpFan1_hHsd4ch1 = uint8(0);
DiagnoseResultStruct.PumpFan2_hHsd4ch2 = uint8(0);

DiagnoseResultStruct.DevicePwr_hHsd5ch1 = uint8(0);
DiagnoseResultStruct.DevicePwr_hHsd5ch2 = uint8(0);

DiagnoseResultStruct.DevicePwr_hHsd6ch1 = uint8(0);
DiagnoseResultStruct.DevicePwr_hHsd6ch2 = uint8(0);

== stateflow chart RBCM_Model/指令报文解码器/Subsystem3/旧模型（放弃）/Chart2 ==
  state close
    output=1;
  state open
    output=0;
  (default) -> close
  close -> open : [input==1]{trigger;}
  open -> close : [input==2]{trigger;}
  data: input input uint8; output output uint32
  events: trigger output FUNCTION_CALL_EVENT

== matlab function RBCM_Model/HSD诊断分析子系统/旧模型/触发器11 ==
  data: y output uint8; counter input uint8; u2 input uint8
  events: fcncall output FUNCTION_CALL_EVENT
function y = fcn(counter,u2)

% 函数内部声明 可持续类型变量 output
persistent i
persistent output  
% 首先要判断persistent声明的变量是否是空
if isempty(i)
    i  = 0;
end
if isempty(output)
    output  = 0;
end

% 自递增
i=i+1;
output=output+1;

%分频计数值溢出
if i>=counter
    %输出值溢出
    if output>=u2
        output=0;
    end

    %输出值
    y = uint8(output);

    %生成触发，触发ADC采集
    fcncall;

    i=0;
else
    y=uint8(output);    %不生成触发
end

end

== matlab function RBCM_Model/HSD诊断分析子系统/触发器2 ==
  data: y output uint8; counter input uint8; u2 input uint8
  events: fcncall output FUNCTION_CALL_EVENT
function y = fcn(counter,u2)

% 函数内部声明 可持续类型变量 output
persistent i
persistent output  
% 首先要判断persistent声明的变量是否是空
if isempty(i)
    i  = 0;
end
if isempty(output)
    output  = 0;
end

% 自递增
i=i+1;
output=output+1;

%分频计数值溢出
if i>=counter
    %输出值溢出
    if output>=u2
        output=0;
    end

    %输出值
    y = uint8(output);

    %生成触发，触发ADC采集
    fcncall;

    i=0;
else
    y=uint8(output);    %不生成触发
end

end

== matlab function RBCM_Model/HSD诊断分析子系统/诊断数据转存单元2 ==
  data: index input uint8; u input uint16; y1 output uint16; y2 output uint16; y3 output uint16; y4 output uint16
function [y1, y2, y3, y4] = fcn2(index, u)

% 函数内部声明 可持续类型变量
persistent Y1 Y2 Y3 Y4
% 首先要判断persistent声明的变量是否是空
if isempty(Y1)
    Y1=uint16(0);
    Y2=uint16(0);
    Y3=uint16(0);
    Y4=uint16(0);
end

if index==0
    y1=u;
    y2=Y2;
    y3=Y3;
    y4=Y4;
elseif index==1
    y1=Y1;
    y2=u;
    y3=Y3;
    y4=Y4;
elseif index==2
    y1=Y1;
    y2=Y2;
    y3=u;
    y4=Y4;
elseif index==3
    y1=Y1;
    y2=Y2;
    y3=Y3;
    y4=u;
else
    y1=Y1;
    y2=Y2;
    y3=Y3;
    y4=Y4;
end

Y1=y1;
Y2=y2;
Y3=y3;
Y4=y4;

end

== matlab function RBCM_Model/HSD诊断分析子系统/错误码转存单元1 ==
  data: index input uint8; u input uint8; y1 output uint8; y2 output uint8; y3 output uint8; y4 output uint8
function [y1, y2, y3, y4] = fcn2(index, u)

% 函数内部声明 可持续类型变量
persistent Y1 Y2 Y3 Y4
% 首先要判断persistent声明的变量是否是空
if isempty(Y1)
    Y1=uint8(0);
    Y2=uint8(0);
    Y3=uint8(0);
    Y4=uint8(0);
end

if index==0
    y1=u;
    y2=Y2;
    y3=Y3;
    y4=Y4;
elseif index==1
    y1=Y1;
    y2=u;
    y3=Y3;
    y4=Y4;
elseif index==2
    y1=Y1;
    y2=Y2;
    y3=u;
    y4=Y4;
elseif index==3
    y1=Y1;
    y2=Y2;
    y3=Y3;
    y4=u;
else
    y1=Y1;
    y2=Y2;
    y3=Y3;
    y4=Y4;
end

Y1=y1;
Y2=y2;
Y3=y3;
Y4=y4;

end

== matlab function RBCM_Model/HSD诊断分析子系统/触发器3 ==
  data: y output uint8; counter input uint8; u2 input uint8
  events: fcncall output FUNCTION_CALL_EVENT
function y = fcn(counter,u2)

% 函数内部声明 可持续类型变量 output
persistent i
persistent output  
% 首先要判断persistent声明的变量是否是空
if isempty(i)
    i  = 0;
end
if isempty(output)
    output  = 0;
end

% 自递增
i=i+1;
output=output+1;

%分频计数值溢出
if i>=counter
    %输出值溢出
    if output>=u2
        output=0;
    end

    %输出值
    y = uint8(output);

    %生成触发，触发ADC采集
    fcncall;

    i=0;
else
    y=uint8(output);    %不生成触发
end

end

== matlab function RBCM_Model/HSD诊断分析子系统/触发器4 ==
  data: y output uint8; counter input uint8; u2 input uint8
  events: fcncall output FUNCTION_CALL_EVENT
function y = fcn(counter,u2)

% 函数内部声明 可持续类型变量 output
persistent i
persistent output  
% 首先要判断persistent声明的变量是否是空
if isempty(i)
    i  = 0;
end
if isempty(output)
    output  = 0;
end

% 自递增
i=i+1;
output=output+1;

%分频计数值溢出
if i>=counter
    %输出值溢出
    if output>=u2
        output=0;
    end

    %输出值
    y = uint8(output);

    %生成触发，触发ADC采集
    fcncall;

    i=0;
else
    y=uint8(output);    %不生成触发
end

end

== matlab function RBCM_Model/HSD诊断分析子系统/诊断数据转存单元3 ==
  data: index input uint8; u input uint16; y1 output uint16; y2 output uint16; y3 output uint16; y4 output uint16
function [y1, y2, y3, y4] = fcn2(index, u)

% 函数内部声明 可持续类型变量
persistent Y1 Y2 Y3 Y4
% 首先要判断persistent声明的变量是否是空
if isempty(Y1)
    Y1=uint16(0);
    Y2=uint16(0);
    Y3=uint16(0);
    Y4=uint16(0);
end

if index==0
    y1=u;
    y2=Y2;
    y3=Y3;
    y4=Y4;
elseif index==1
    y1=Y1;
    y2=u;
    y3=Y3;
    y4=Y4;
elseif index==2
    y1=Y1;
    y2=Y2;
    y3=u;
    y4=Y4;
elseif index==3
    y1=Y1;
    y2=Y2;
    y3=Y3;
    y4=u;
else
    y1=Y1;
    y2=Y2;
    y3=Y3;
    y4=Y4;
end

Y1=y1;
Y2=y2;
Y3=y3;
Y4=y4;

end

== matlab function RBCM_Model/HSD诊断分析子系统/诊断数据转存单元4 ==
  data: index input uint8; u input uint16; y1 output uint16; y2 output uint16; y3 output uint16; y4 output uint16
function [y1, y2, y3, y4] = fcn2(index, u)

% 函数内部声明 可持续类型变量
persistent Y1 Y2 Y3 Y4
% 首先要判断persistent声明的变量是否是空
if isempty(Y1)
    Y1=uint16(0);
    Y2=uint16(0);
    Y3=uint16(0);
    Y4=uint16(0);
end

if index==0
    y1=u;
    y2=Y2;
    y3=Y3;
    y4=Y4;
elseif index==1
    y1=Y1;
    y2=u;
    y3=Y3;
    y4=Y4;
elseif index==2
    y1=Y1;
    y2=Y2;
    y3=u;
    y4=Y4;
elseif index==3
    y1=Y1;
    y2=Y2;
    y3=Y3;
    y4=u;
else
    y1=Y1;
    y2=Y2;
    y3=Y3;
    y4=Y4;
end

Y1=y1;
Y2=y2;
Y3=y3;
Y4=y4;

end
